simulink library "Lib_Turbo_FlowPathChar_TMATS_org"  (Simulink 10.0)
settings: Solver=ode45  StartTime=0.0  StopTime=10.0  RelTol=1e-3  EnableMultiTasking=on
libraries: Lib_Thermo_Temp2Enth_TMATS x1
Description:
  | Thomas Modules
settings Model: Creator=jwchapm2  LastModifiedBy=annonymous

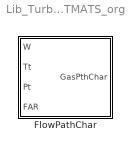
== system Lib_Turbo_FlowPathChar_TMATS_org ==
  FlowPathChar : Subsystem  mask(T-MATS: Flow Path Characteristics Library Block){}
      mask help: This block creates a flow path characteristics bus for input into the system.
      mask Help: web(which('Turbo_TMATS_FPC.html'),'-helpbrowser')

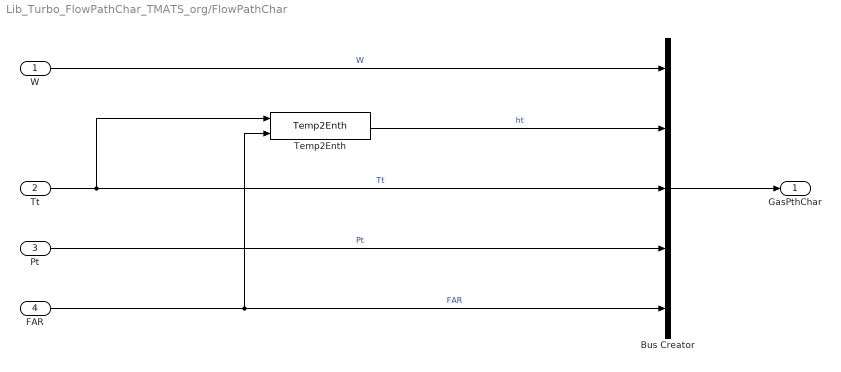
== system Lib_Turbo_FlowPathChar_TMATS_org/FlowPathChar ==
  W : Inport
  Tt : Inport  Port=2
  Pt : Inport  Port=3
  FAR : Inport  Port=4
  Bus Creator : BusCreator  Inputs=5
  Temp2Enth : Lib_Thermo_Temp2Enth_TMATS/Temp2Enth
  GasPthChar : Outport
  wires:
  W/1 -> Bus Creator/1  "W"
  Pt/1 -> Bus Creator/4  "Pt"
  FAR/1 -> Temp2Enth/2, Bus Creator/5  "FAR"
  Bus Creator/1 -> GasPthChar/1
  Tt/1 -> Temp2Enth/1, Bus Creator/3  "Tt"
  Temp2Enth/1 -> Bus Creator/2  "ht"
